simulink model "Id_project"  (R2015a)
settings: Solver=ode45  StartTime=0.0  StopTime=10.0  RelTol=1e-3
undefined symbols (not defined in the file): sigbuilder_block
settings Model: Creator=hp  LastModifiedBy=hp

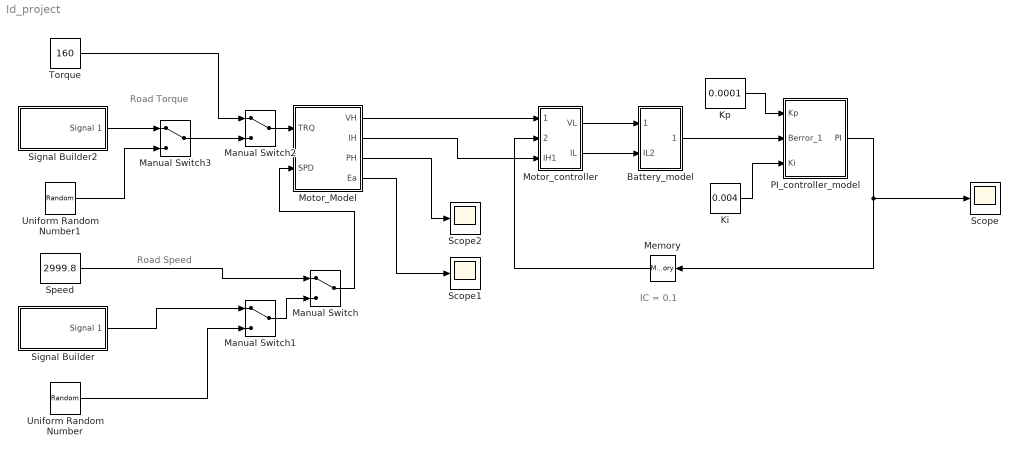
== system Id_project ==
  note: Road Speed
  note: Road Torque
  note: IC = 0.1
  Battery_model : Subsystem
  Ki : Constant  Value=0.004
  Kp : Constant  Value=0.0001
  Manual Switch{,1..3} (4 alike) : ManualSwitch
  Memory : Memory  X0=0.1
  Motor_Model : Subsystem
  Motor_controller : Subsystem
  PI_controller_model : Subsystem
  Scope : Scope
      settings: YMin=-0.5  YMax=2
  Scope1 : Scope
      settings: TimeRange=10  YMin=540  YMax=542.5
  Scope2 : Scope
      settings: SaveName=ScopeData2
  Signal Builder : Subsystem  Tag=STV Subsys  LoadFcn=sigbuilder_block('load');  StartFcn=sigbuilder_block('start');  StopFcn=sigbuilder_block('stop');  ClipboardFcn=sigbuilder_block('clipboard');  mask(Sigbuilder block){}
      mask help: Simulink:masks:SigbuilderBlock_MD
      mask init:
      | if ~strcmp(get_param(bdroot(gcbh),'SimulationStatus'),'stopped') tuvar = sigbuilder_block('maskInit'); end
      settings: CopyFcn=sigbuilder_block('copy');  DeleteFcn=sigbuilder_block('delete');  ModelCloseFcn=sigbuilder_block('modelClose');  PreSaveFcn=sigbuilder_block('preSave');  PauseFcn=sigbuilder_block('pause');  ContinueFcn=sigbuilder_block('continue');  NameChangeFcn=sigbuilder_block('namechange');  OpenFcn=sigbuilder_block('open',[437.6 199.2 550.4 400 ]);  CloseFcn=sigbuilder_block('close');
      mask Display: plot(0, 0, 100, 100,[2, 2, 32, 32, 2], [68, 8, 8, 68, 68],[32, 2], [38, 38], [32, 19, 2],[53, 60, 44], [32, 17, 17, 2],[16, 16, 31, 31]);txt = getActiveGroup(gcbh);text(2, 100, txt,'verticalAlignment', 'top');
  Signal Builder2 : Subsystem  Tag=STV Subsys  LoadFcn=sigbuilder_block('load');  StartFcn=sigbuilder_block('start');  StopFcn=sigbuilder_block('stop');  ClipboardFcn=sigbuilder_block('clipboard');  mask(Sigbuilder block){}
      mask help: Simulink:masks:SigbuilderBlock_MD
      mask init:
      | if ~strcmp(get_param(bdroot(gcbh),'SimulationStatus'),'stopped') tuvar = sigbuilder_block('maskInit'); end
      settings: CopyFcn=sigbuilder_block('copy');  DeleteFcn=sigbuilder_block('delete');  ModelCloseFcn=sigbuilder_block('modelClose');  PreSaveFcn=sigbuilder_block('preSave');  PauseFcn=sigbuilder_block('pause');  ContinueFcn=sigbuilder_block('continue');  NameChangeFcn=sigbuilder_block('namechange');  OpenFcn=sigbuilder_block('open',[437.6 199.2 550.4 400 ]);  CloseFcn=sigbuilder_block('close');
      mask Display: plot(0, 0, 100, 100,[2, 2, 32, 32, 2], [68, 8, 8, 68, 68],[32, 2], [38, 38], [32, 19, 2],[53, 60, 44], [32, 17, 17, 2],[16, 16, 31, 31]);txt = getActiveGroup(gcbh);text(2, 100, txt,'verticalAlignment', 'top');
  Speed : Constant  Value=2999.8
  Torque : Constant  Value=160
  Uniform Random Number : UniformRandomNumber  Minimum=1500  Maximum=3000  SampleTime=0.1
  Uniform Random Number1 : UniformRandomNumber  Minimum=-50  Maximum=200  SampleTime=0.1
  wires:
  Motor_Model/1(VH) -> Motor_controller/1(VH1)
  Motor_Model/2(IH) -> Motor_controller/3(IH1)
  Motor_Model/3(PH) -> Scope2/1
  Motor_Model/4(Ea) -> Scope1/1
  Memory/1 -> Motor_controller/2(Kval)
  Motor_controller/1(VL) -> Battery_model/1(VL2)
  Motor_controller/2(IL) -> Battery_model/2(IL2)
  Battery_model/1(Berror) -> PI_controller_model/2(Berror_1)
  PI_controller_model/1(PI) -> Scope/1, Memory/1
  Ki/1 -> PI_controller_model/3(Ki)
  Kp/1 -> PI_controller_model/1(Kp)
  Manual Switch/1 -> Motor_Model/2(SPD)
  Manual Switch1/1 -> Manual Switch/2
  Speed/1 -> Manual Switch/1
  Signal Builder/1(Signal 1) -> Manual Switch1/1
  Uniform Random Number/1 -> Manual Switch1/2
  Manual Switch3/1 -> Manual Switch2/2
  Manual Switch2/1 -> Motor_Model/1(TRQ)
  Torque/1 -> Manual Switch2/1
  Signal Builder2/1(Signal 1) -> Manual Switch3/1
  Uniform Random Number1/1 -> Manual Switch3/2

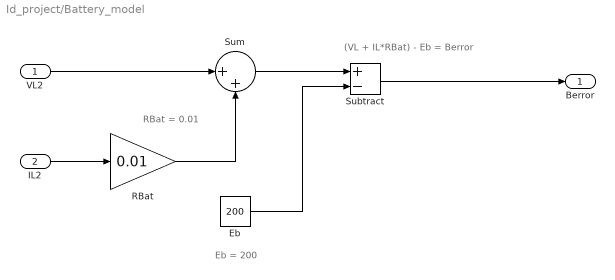
== system Id_project/Battery_model ==
  note: (VL + IL*RBat) - Eb = Berror
  note: Eb = 200
  note: RBat = 0.01
  VL2 : Inport
  IL2 : Inport  Port=2
  Eb : Constant  Value=200
  RBat : Gain  Gain=0.01
  Subtract : Sum  Inputs=+-
  Sum : Sum  Inputs=|++
  Berror : Outport
  wires:
  RBat/1 -> Sum/2
  Sum/1 -> Subtract/1
  IL2/1 -> RBat/1
  VL2/1 -> Sum/1
  Eb/1 -> Subtract/2
  Subtract/1 -> Berror/1

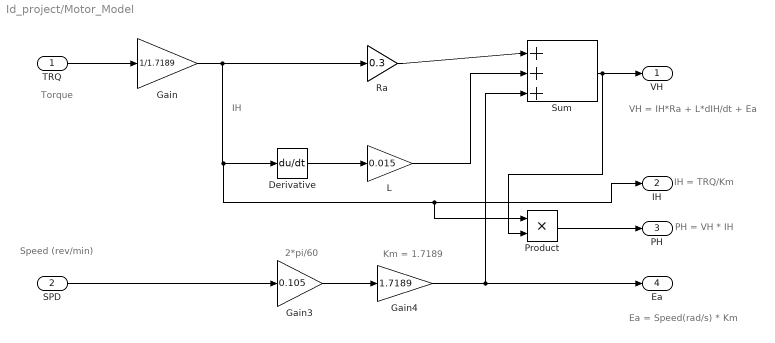
== system Id_project/Motor_Model ==
  note: IH
  note: Ea = Speed(rad/s) * Km
  note: PH = VH * IH
  note: IH = TRQ/Km
  note: VH = IH*Ra + L*dIH/dt + Ea
  note: Km = 1.7189
  note: 2*pi/60
  note: Torque
  note: Speed (rev/min)
  TRQ : Inport
  SPD : Inport  Port=2
  Derivative : Derivative
  Gain : Gain  Gain=1/1.7189
  Gain3 : Gain  Gain=0.105
  Gain4 : Gain  Gain=1.7189
  L : Gain  Gain=0.015
  Product : Product
  Ra : Gain  Gain=0.3
  Sum : Sum  Inputs=|+++
  VH : Outport
  IH : Outport  Port=2
  PH : Outport  Port=3
  Ea : Outport  Port=4
  wires:
  TRQ/1 -> Gain/1
  Sum/1 -> VH/1, Product/2
  L/1 -> Sum/2
  Gain3/1 -> Gain4/1
  Gain4/1 -> Ea/1, Sum/3
  Gain/1 -> IH/1, Product/1, Derivative/1, Ra/1
  SPD/1 -> Gain3/1
  Product/1 -> PH/1
  Derivative/1 -> L/1
  Ra/1 -> Sum/1

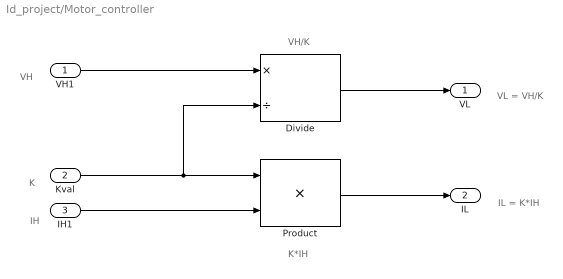
== system Id_project/Motor_controller ==
  note: IL = K*IH
  note: VL = VH/K
  note: K*IH
  note: IH
  note: K
  note: VH
  note: VH/K
  VH1 : Inport
  Kval : Inport  Port=2
  IH1 : Inport  Port=3
  Divide : Product  Inputs=*/
  Product : Product
  VL : Outport
  IL : Outport  Port=2
  wires:
  VH1/1 -> Divide/1
  Product/1 -> IL/1
  Divide/1 -> VL/1
  Kval/1 -> Divide/2, Product/1
  IH1/1 -> Product/2

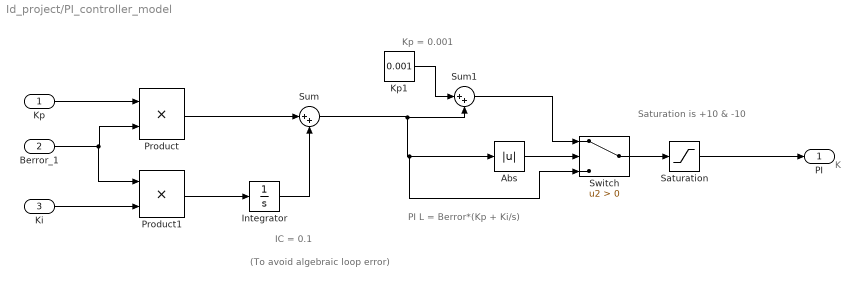
== system Id_project/PI_controller_model ==
  note: K
  note: Saturation is +10 & -10
  note: PI
      | L = Berror*(Kp + Ki/s)
  note: (To avoid algebraic loop error)
  note: IC = 0.1
  note: Kp = 0.001
  Kp : Inport
  Berror_1 : Inport  Port=2
  Ki : Inport  Port=3
  Abs : Abs
  Integrator : Integrator  InitialCondition=0.1
  Kp1 : Constant  Value=0.001
  Product : Product
  Product1 : Product
  Saturation : Saturate  UpperLimit=+10  LowerLimit=-10
  Sum : Sum  Inputs=|++
  Sum1 : Sum  Inputs=|++
  Switch : Switch  Criteria=u2 > Threshold
  PI : Outport
  wires:
  Switch/1 -> Saturation/1
  Saturation/1 -> PI/1
  Kp1/1 -> Sum1/1
  Product1/1 -> Integrator/1
  Sum/1 -> Sum1/2, Switch/3, Abs/1
  Abs/1 -> Switch/2
  Product/1 -> Sum/1
  Integrator/1 -> Sum/2
  Sum1/1 -> Switch/1
  Kp/1 -> Product/1
  Ki/1 -> Product1/2
  Berror_1/1 -> Product1/1, Product/2

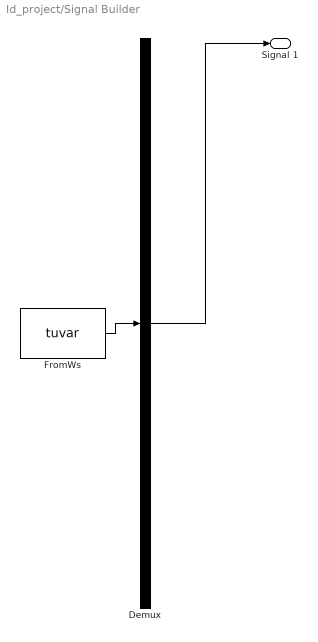
== system Id_project/Signal Builder ==
  Demux : Demux  Tag=STV Demux  Outputs=1
  FromWs : FromWorkspace  Tag=STV FromWs  VariableName=tuvar  SampleTime=0
      SigBuilderData=|
      | common.afterFinalStr = 'Extrapolate'
      | common.sampleTime = 0
      | dataSet.timeRange = [0 10]
      | dataSet.name = 'Group 1'
      | sbobj.Groups.Name = 'Group 1'
      | sbobj.Groups.Signals.Name = 'Signal 1'
      | sbobj.Groups.Signals.XData = [0 0.68 0.68 6 10]
      | sbobj.Groups.Signals.YData = [0 0 2000 3000 0]
  Signal 1 : Outport  Tag=STV Outport
  wires:
  Demux/1 -> Signal 1/1
  FromWs/1 -> Demux/1

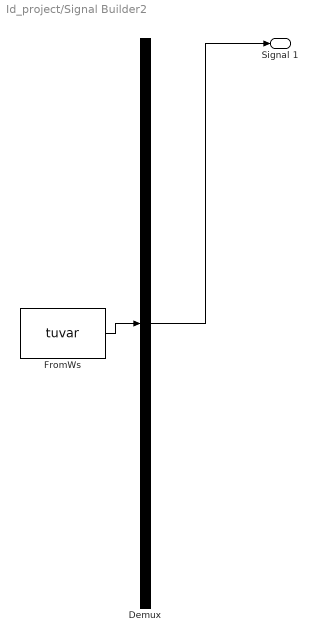
== system Id_project/Signal Builder2 ==
  Demux : Demux  Tag=STV Demux  Outputs=1
  FromWs : FromWorkspace  Tag=STV FromWs  VariableName=tuvar  SampleTime=0
      SigBuilderData=|
      | common.afterFinalStr = 'Extrapolate'
      | common.sampleTime = 0
      | dataSet.timeRange = [0 10]
      | dataSet.name = 'Group 1'
      | sbobj.Groups.Name = 'Group 1'
      | sbobj.Groups.Signals.Name = 'Signal 1'
      | sbobj.Groups.Signals.XData = [0 0.68 0.68 6 10]
      | sbobj.Groups.Signals.YData = [0 0 50 250 -106]
  Signal 1 : Outport  Tag=STV Outport
  wires:
  FromWs/1 -> Demux/1
  Demux/1 -> Signal 1/1
